simulink model "physicsPos"  (R2016b)
settings: Solver=ode45  StartTime=0.0  StopTime=10.0  RelTol=1e-3  EnableMultiTasking=on
undefined symbols (not defined in the file or in its folder): Kd, M
settings Model: Creator=Cassandra  LastModifiedBy=Cassandra
settings DataIOCC: LimitDataPoints=on  SaveFormat=Array
settings OptimizationCC: LifeSpan=inf
settings DebuggingCC: SFUnexpectedBacktrackingDiag=warning  SFNoUnconditionalDefaultTransitionDiag=warning  SFExecutionAtInitializationDiag=none
settings HardwareCC: ProdBitPerPointer=32  ProdBitPerSizeT=32  ProdBitPerPtrDiffT=32  ProdLargestAtomicFloat=None  ProdIntDivRoundTo=Undefined  ProdEndianess=Unspecified  ProdWordSize=32  ProdHWDeviceType=32-bit Generic
settings ModelReferenceCC: PropagateSignalLabelsOutOfModel=off
settings GRTTargetCC: TargetLangStandard=C89/C90 (ANSI)  GeneratePreprocessorConditionals=Disable all
settings ConfigComp: CovMetricSettings=dw  CovHtmlReporting=on  CovSaveCumulativeToWorkspaceVar=on  CovSaveSingleToWorkspaceVar=on  CovExternalEMLEnable=off

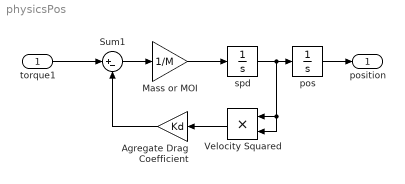
== system physicsPos ==
  torque1 : Inport
  Agregate Drag Coefficient : Gain  Gain=Kd
  Mass or MOI : Gain  Gain=1/M
  Sum1 : Sum  Inputs=|+-
  Velocity Squared : Product
  pos : Integrator
  spd : Integrator
  position : Outport
  wires:
  Mass or MOI/1 -> spd/1
  spd/1 -> Velocity Squared/2, Velocity Squared/1, pos/1
  Sum1/1 -> Mass or MOI/1
  torque1/1 -> Sum1/1
  pos/1 -> position/1
  Velocity Squared/1 -> Agregate Drag Coefficient/1
  Agregate Drag Coefficient/1 -> Sum1/2
